simulink library "ammclib_bam_s32k11x"  (Simulink 9.0)
settings: Solver=ode45  StartTime=0.0  StopTime=10.0  RelTol=1e-3
undefined symbols (not defined in the file): f16A1, f16A2, f16B0, f16B1, f16B2, f16C1, f16CC1, f16CC1sc, f16CC1sc_D, f16CC1sc_Q, f16CC1scD, f16CC1scQ, f16CC2, f16CC2sc, f16CC2sc_D, f16CC2sc_Q, f16CC2scD, f16CC2scQ, f16DerivGain, f16EGain, f16FiltCoef, f16HystOff, f16HystOn, f16IGain, f16IntegGain, f16IntegGainFW, f16IntegGainQ, f16Kd, f16Kq, f16Limit, f16LowerLim, f16LowerLimit_D, f16LowerLimit_Q, f16ModIndex, f16OutValOff, f16OutValOn, f16PropGain, f16PropGainFW, f16PropGainQ, f16RampDown, f16RampUp, f16UGain, f16UpperLim, f16UpperLimit, f16UpperLimit_D, f16UpperLimit_Q, f16WIGain, f32A1, f32A2, f32B0, f32B1, f32B2, f32C1, f32CC1, f32CC1sc, f32CC1sc_D, f32CC1sc_Q, f32CC1scD, f32CC1scQ, f32CC2 ... (+71)
(part 5 of 7)

== system ammclib_bam_s32k11x/GFLIB/bam_f32/GFLIB_ControllerPIDpAW_F32 ==
  note: ---------------------------------------------------------------------------------------------------------------------------------------------------------------------------------------------------
  f32InErr : Inport
  f32UpperLimit : Inport  Port=2
  f32LowerLimit : Inport  Port=3
  Delay : Delay  DelayLength=1  InitialCondition=0
  Delay1 : Delay  DelayLength=1  InitialCondition=0
  Delay2 : Delay  DelayLength=1  InitialCondition=0
  GFLIB_ControllerPIDpAW_SF : S-Function  FunctionName=GFLIB_ControllerPIDpAW_SF_F32  Parameters=f32PropGain,s16PropGainShift,f32IntegGain,s16IntegGainShift,f32DerivGain,s16DerivGainShift,f32FiltCoef  SFunctionDeploymentMode=off  EnableBusSupport=off
  copyright : Subsystem
      mask Display: text(10,90,'FILE:');text(10,75,'DESRIPTION:');text(10,60,'COPYRIGHT:');text(10,45,'VERSION:');text(10,30,'DATE:')
  copyright2 : Subsystem
      mask Display: text(10,90,'GFLIB_ControllerPIDpAW_BAM_F32.mdl');text(10,75,'Parallel form of a standard PID controller with implemented anti-windup.');text(10,60,'NXP');text(10,45,'0.1');text(10,30,'21-Nov-2018');
  logo : Subsystem
      mask Display: image(imread('logo.jpg'))
  f32Out : Outport
  u16LimitFlag : Outport  Port=2
  wires:
  f32InErr/1 -> GFLIB_ControllerPIDpAW_SF/1
  f32UpperLimit/1 -> GFLIB_ControllerPIDpAW_SF/2
  f32LowerLimit/1 -> GFLIB_ControllerPIDpAW_SF/3
  Delay2/1 -> GFLIB_ControllerPIDpAW_SF/4
  Delay1/1 -> GFLIB_ControllerPIDpAW_SF/5
  Delay/1 -> GFLIB_ControllerPIDpAW_SF/6
  GFLIB_ControllerPIDpAW_SF/1 -> f32Out/1
  GFLIB_ControllerPIDpAW_SF/2 -> u16LimitFlag/1
  GFLIB_ControllerPIDpAW_SF/3 -> Delay2/1
  GFLIB_ControllerPIDpAW_SF/4 -> Delay1/1
  GFLIB_ControllerPIDpAW_SF/5 -> Delay/1

== system ammclib_bam_s32k11x/GFLIB/bam_f32/GFLIB_ControllerPIpAW_F32 ==
  note: ---------------------------------------------------------------------------------------------------------------------------------------------------------------------------------------------------
  f32InErr : Inport
  f32UpperLimit : Inport  Port=2
  f32LowerLimit : Inport  Port=3
  GFLIB_ControllerPIpAW_SF : S-Function  FunctionName=GFLIB_ControllerPIpAW_SF_F32  Parameters=f32PropGain,s16PropGainShift,f32IntegGain,s16IntegGainShift  SFunctionDeploymentMode=off  EnableBusSupport=off
  Unit_Delay_f32InK_1 : Delay  DelayLength=1  InitialCondition=0
  Unit_Delay_f32IntegPartK_1 : Delay  DelayLength=1  InitialCondition=0
  copyright : Subsystem
      mask Display: text(10,90,'FILE:');text(10,75,'DESRIPTION:');text(10,60,'COPYRIGHT:');text(10,45,'VERSION:');text(10,30,'DATE:')
  copyright2 : Subsystem
      mask Display: text(10,90,'GFLIB_ControllerPIpAW_BAM_F32.mdl');text(10,75,'Parallel form of a standard PI controller with implemented anti-windup.');text(10,60,'NXP');text(10,45,'0.1');text(10,30,'12-Jun-2015');
  logo : Subsystem
      mask Display: image(imread('logo.jpg'))
  f32Out : Outport
  u16LimitFlag : Outport  Port=2
  wires:
  GFLIB_ControllerPIpAW_SF/2 -> u16LimitFlag/1
  GFLIB_ControllerPIpAW_SF/1 -> f32Out/1
  f32LowerLimit/1 -> GFLIB_ControllerPIpAW_SF/3
  f32UpperLimit/1 -> GFLIB_ControllerPIpAW_SF/2
  f32InErr/1 -> GFLIB_ControllerPIpAW_SF/1
  Unit_Delay_f32IntegPartK_1/1 -> GFLIB_ControllerPIpAW_SF/5
  Unit_Delay_f32InK_1/1 -> GFLIB_ControllerPIpAW_SF/4
  GFLIB_ControllerPIpAW_SF/4 -> Unit_Delay_f32IntegPartK_1/1
  GFLIB_ControllerPIpAW_SF/3 -> Unit_Delay_f32InK_1/1

== system ammclib_bam_s32k11x/GFLIB/bam_f32/GFLIB_ControllerPIp_F32 ==
  note: ---------------------------------------------------------------------------------------------------------------------------------------------------------------------------------------------------
  f32InErr : Inport
  GFLIB_ControllerPIp_SF : S-Function  FunctionName=GFLIB_ControllerPIp_SF_F32  Parameters=f32PropGain,s16PropGainShift,f32IntegGain,s16IntegGainShift  SFunctionDeploymentMode=off  EnableBusSupport=off
  Unit_Delay_f32InIntegPartK_1 : UnitDelay  SampleTime=-1
  Unit_Delay_f32InK_1 : UnitDelay  SampleTime=-1
  copyright : Subsystem
      mask Display:
      | text(10,90,'FILE:');text(10,75,'DESRIPTION:')
      | text(10,60,'COPYRIGHT:')
      | text(10,45,'VERSION:')
      | text(10,30,'DATE:')
  copyright2 : Subsystem
      mask Display:
      | text(10,90,'GFLIB_ControllerPIp_BAM_F32.mdl');text(10,75,'Parallel form of a standard PI controller without implemented anti-windup.');text(10,60,'NXP')
      | text(10,45,'0.1');text(10,30,'20-Jan-2012');
  logo : Subsystem
      mask Display: image(imread('logo.jpg'))
  f32Out : Outport
  wires:
  GFLIB_ControllerPIp_SF/1 -> f32Out/1
  f32InErr/1 -> GFLIB_ControllerPIp_SF/1
  GFLIB_ControllerPIp_SF/3 -> Unit_Delay_f32InIntegPartK_1/1
  Unit_Delay_f32InIntegPartK_1/1 -> GFLIB_ControllerPIp_SF/3
  Unit_Delay_f32InK_1/1 -> GFLIB_ControllerPIp_SF/2
  GFLIB_ControllerPIp_SF/2 -> Unit_Delay_f32InK_1/1

== system ammclib_bam_s32k11x/GFLIB/bam_f32/GFLIB_ControllerPIrAW_F32 ==
  note: ---------------------------------------------------------------------------------------------------------------------------------------------------------------------------------------------------
  f32InErr : Inport
  f32UpperLimit : Inport  Port=2
  f32LowerLimit : Inport  Port=3
  GFLIB_ControllerPIrAW_SF : S-Function  FunctionName=GFLIB_ControllerPIrAW_SF_F32  Parameters=f32CC1,f32CC2,u16NShift  SFunctionDeploymentMode=off  EnableBusSupport=off
  Unit_Delay_f32Acc : Delay  DelayLength=1  InitialCondition=0
  Unit_Delay_f32InErrK1 : Delay  DelayLength=1  InitialCondition=0
  copyright : Subsystem
      mask Display: text(10,90,'FILE:');text(10,75,'DESRIPTION:');text(10,60,'COPYRIGHT:');text(10,45,'VERSION:');text(10,30,'DATE:')
  copyright2 : Subsystem
      mask Display: text(10,90,'GFLIB_ControllerPIrAW_BAM_F32.mdl');text(10,75,'Recurrent form of a standard PI controller with implemented anti-windup functionality.');text(10,60,'NXP');text(10,45,'0.1');text(10,30,'12-Jun-2015');
  logo : Subsystem
      mask Display: image(imread('logo.jpg'))
  f32Out : Outport
  wires:
  GFLIB_ControllerPIrAW_SF/1 -> f32Out/1
  f32LowerLimit/1 -> GFLIB_ControllerPIrAW_SF/3
  f32UpperLimit/1 -> GFLIB_ControllerPIrAW_SF/2
  f32InErr/1 -> GFLIB_ControllerPIrAW_SF/1
  GFLIB_ControllerPIrAW_SF/3 -> Unit_Delay_f32InErrK1/1
  GFLIB_ControllerPIrAW_SF/2 -> Unit_Delay_f32Acc/1
  Unit_Delay_f32InErrK1/1 -> GFLIB_ControllerPIrAW_SF/5
  Unit_Delay_f32Acc/1 -> GFLIB_ControllerPIrAW_SF/4

== system ammclib_bam_s32k11x/GFLIB/bam_f32/GFLIB_ControllerPIr_F32 ==
  note: ---------------------------------------------------------------------------------------------------------------------------------------------------------------------------------------------------
  f32InErr : Inport
  GFLIB_ControllerPIr_SF : S-Function  FunctionName=GFLIB_ControllerPIr_SF_F32  Parameters=f32CC1,f32CC2,u16NShift  SFunctionDeploymentMode=off  EnableBusSupport=off
  Unit_Delay_f32AccIn : UnitDelay  SampleTime=-1
  Unit_Delay_f32InErrK_1 : UnitDelay  SampleTime=-1
  copyright : Subsystem
      mask Display:
      | text(10,90,'FILE:');text(10,75,'DESRIPTION:')
      | text(10,60,'COPYRIGHT:')
      | text(10,45,'VERSION:')
      | text(10,30,'DATE:')
  copyright2 : Subsystem
      mask Display:
      | text(10,90,'GFLIB_ControllerPIr_BAM_F32.mdl');text(10,75,'Recurrent form of a standard PI controller without implemented anti-windup.');text(10,60,'NXP')
      | text(10,45,'0.1');text(10,30,'20-Jan-2012');
  logo : Subsystem
      mask Display: image(imread('logo.jpg'))
  f32Out : Outport
  wires:
  GFLIB_ControllerPIr_SF/1 -> f32Out/1
  f32InErr/1 -> GFLIB_ControllerPIr_SF/1
  Unit_Delay_f32InErrK_1/1 -> GFLIB_ControllerPIr_SF/3
  Unit_Delay_f32AccIn/1 -> GFLIB_ControllerPIr_SF/2
  GFLIB_ControllerPIr_SF/3 -> Unit_Delay_f32InErrK_1/1
  GFLIB_ControllerPIr_SF/2 -> Unit_Delay_f32AccIn/1

== system ammclib_bam_s32k11x/GFLIB/bam_f32/GFLIB_Cos_F32 ==
  note: ---------------------------------------------------------------------------------------------------------------------------------------------------------------------------------------------------
  f32In : Inport
  GFLIB_Cos_SF : S-Function  FunctionName=GFLIB_Cos_SF_F32  SFunctionDeploymentMode=off  EnableBusSupport=off
  copyright : Subsystem
      mask Display: text(10,90,'FILE:');text(10,75,'DESRIPTION:')text(10,60,'COPYRIGHT:')text(10,45,'VERSION:')text(10,30,'DATE:')
  copyright2 : Subsystem
      mask Display: text(10,90,'GFLIB_Cos_BAM_F32.mdl');text(10,75,'Cosine transformation');text(10,60,'NXP')text(10,45,'0.1');text(10,30,'13-Sep-2011');
  logo : Subsystem
      mask Display: image(imread('logo.jpg'))
  f32Out : Outport
  wires:
  GFLIB_Cos_SF/1 -> f32Out/1
  f32In/1 -> GFLIB_Cos_SF/1

== system ammclib_bam_s32k11x/GFLIB/bam_f32/GFLIB_Hyst_F32 ==
  note: ---------------------------------------------------------------------------------------------------------------------------------------------------------------------------------------------------
  f32In : Inport
  GFLIB_Hyst_SF_F32 : S-Function  FunctionName=GFLIB_Hyst_SF_F32  Parameters=f32HystOn,f32HystOff,f32OutValOn,f32OutValOff  SFunctionDeploymentMode=off  EnableBusSupport=off
  Unit_Delay_f32InState : UnitDelay  SampleTime=-1
  copyright : Subsystem
      mask Display:
      | text(10,90,'FILE:');text(10,75,'DESRIPTION:')
      | text(10,60,'COPYRIGHT:')
      | text(10,45,'VERSION:')
      | text(10,30,'DATE:')
  copyright2 : Subsystem
      mask Display:
      | text(10,90,'GFLIB_Hyst_BAM_F32.mdl');text(10,75,'Hysteresis function.');text(10,60,'NXP')
      | text(10,45,'0.1');text(10,30,'09-Apr-2014');
  logo : Subsystem
      mask Display: image(imread('logo.jpg'))
  f32Out : Outport
  wires:
  GFLIB_Hyst_SF_F32/1 -> f32Out/1
  f32In/1 -> GFLIB_Hyst_SF_F32/1
  Unit_Delay_f32InState/1 -> GFLIB_Hyst_SF_F32/2
  GFLIB_Hyst_SF_F32/2 -> Unit_Delay_f32InState/1

== system ammclib_bam_s32k11x/GFLIB/bam_f32/GFLIB_IntegratorTR_F32 ==
  note: ---------------------------------------------------------------------------------------------------------------------------------------------------------------------------------------------------
  f32In : Inport
  GFLIB_IntegratorTR_SF : S-Function  FunctionName=GFLIB_IntegratorTR_SF_F32  Parameters=f32C1,u16NShift  SFunctionDeploymentMode=off  EnableBusSupport=off
  Unit_Delay_f32InAcc : UnitDelay  SampleTime=-1
  Unit_Delay_f32InK_1 : UnitDelay  SampleTime=-1
  copyright : Subsystem
      mask Display:
      | text(10,90,'FILE:');text(10,75,'DESRIPTION:')
      | text(10,60,'COPYRIGHT:')
      | text(10,45,'VERSION:')
      | text(10,30,'DATE:')
  copyright2 : Subsystem
      mask Display:
      | text(10,90,'GFLIB_IntegratorTR_BAM_F32.mdl');text(10,75,'Discrete integrator transformed from linear model using Billinear (trapezoidal) transformation.');text(10,60,'NXP')
      | text(10,45,'0.1');text(10,30,'16-Jan-2012');
  logo : Subsystem
      mask Display: image(imread('logo.jpg'))
  f32Out : Outport
  wires:
  GFLIB_IntegratorTR_SF/1 -> f32Out/1
  f32In/1 -> GFLIB_IntegratorTR_SF/1
  GFLIB_IntegratorTR_SF/3 -> Unit_Delay_f32InK_1/1
  Unit_Delay_f32InK_1/1 -> GFLIB_IntegratorTR_SF/3
  Unit_Delay_f32InAcc/1 -> GFLIB_IntegratorTR_SF/2
  GFLIB_IntegratorTR_SF/2 -> Unit_Delay_f32InAcc/1

== system ammclib_bam_s32k11x/GFLIB/bam_f32/GFLIB_Limit_F32 ==
  note: ---------------------------------------------------------------------------------------------------------------------------------------------------------------------------------------------------
  f32In : Inport
  GFLIB_Limit_SF_F32 : S-Function  FunctionName=GFLIB_Limit_SF_F32  Parameters=f32UpperLimit,f32LowerLim  SFunctionDeploymentMode=off  EnableBusSupport=off
  copyright : Subsystem
      mask Display:
      | text(10,90,'FILE:');text(10,75,'DESRIPTION:')
      | text(10,60,'COPYRIGHT:')
      | text(10,45,'VERSION:')
      | text(10,30,'DATE:')
      | text(10,15,'AUTHOR:')
  copyright2 : Subsystem
      mask Display:
      | text(10,90,'GFLIB_Limit_BAM_F32.mdl');text(10,75,'Limit function');text(10,60,'NXP')
      | text(10,45,'0.1');text(10,30,'03-Jul-2011');text(10,15,'');
  logo : Subsystem
      mask Display: image(imread('logo.jpg'))
  f32Out : Outport
  wires:
  GFLIB_Limit_SF_F32/1 -> f32Out/1
  f32In/1 -> GFLIB_Limit_SF_F32/1

== system ammclib_bam_s32k11x/GFLIB/bam_f32/GFLIB_LowerLimit_F32 ==
  note: ---------------------------------------------------------------------------------------------------------------------------------------------------------------------------------------------------
  f32In : Inport
  GFLIB_LowerLimit_SF_F32 : S-Function  FunctionName=GFLIB_LowerLimit_SF_F32  Parameters=f32LowerLim  SFunctionDeploymentMode=off  EnableBusSupport=off
  copyright : Subsystem
      mask Display:
      | text(10,90,'FILE:');text(10,75,'DESRIPTION:')
      | text(10,60,'COPYRIGHT:')
      | text(10,45,'VERSION:')
      | text(10,30,'DATE:')
  copyright2 : Subsystem
      mask Display:
      | text(10,90,'GFLIB_LowerLimit_BAM_F32.mdl');text(10,75,'Lower limit function.');text(10,60,'Freescale')
      | text(10,45,'0.1');text(10,30,'13-Sep-2011');
  logo : Subsystem
      mask Display: image(imread('logo.jpg'))
  f32Out : Outport
  wires:
  GFLIB_LowerLimit_SF_F32/1 -> f32Out/1
  f32In/1 -> GFLIB_LowerLimit_SF_F32/1

== system ammclib_bam_s32k11x/GFLIB/bam_f32/GFLIB_Lut1D_F32 ==
  note: ---------------------------------------------------------------------------------------------------------------------------------------------------------------------------------------------------
  f32In : Inport
  GFLIB_Lut1D_SF : S-Function  FunctionName=GFLIB_Lut1D_SF_F32  Parameters=u32ShamOffset,pf32Table,s32MidIdx  SFunctionDeploymentMode=off  EnableBusSupport=off
  copyright : Subsystem
      mask Display:
      | text(10,90,'FILE:');text(10,75,'DESRIPTION:')
      | text(10,60,'COPYRIGHT:')
      | text(10,45,'VERSION:')
      | text(10,30,'DATE:')
  copyright2 : Subsystem
      mask Display:
      | text(10,90,'GFLIB_Lut1D_BAM_F32.mdl');text(10,75,'One dimensional Look-up table function');text(10,60,'Freescale')
      | text(10,45,'0.1');text(10,30,'17-Jun-2013');
  logo : Subsystem
      mask Display: image(imread('logo.jpg'))
  f32Out : Outport
  wires:
  f32In/1 -> GFLIB_Lut1D_SF/1
  GFLIB_Lut1D_SF/1 -> f32Out/1

== system ammclib_bam_s32k11x/GFLIB/bam_f32/GFLIB_Lut2D_F32 ==
  note: ---------------------------------------------------------------------------------------------------------------------------------------------------------------------------------------------------
  f32In1 : Inport
  f32In2 : Inport  Port=2
  GFLIB_Lut2D_SF : S-Function  FunctionName=GFLIB_Lut2D_SF_F32  Parameters=u32ShamOffset1,u32ShamOffset2,pf32Table,s32MidIdx  SFunctionDeploymentMode=off  EnableBusSupport=off
  copyright : Subsystem
      mask Display:
      | text(10,90,'FILE:');text(10,75,'DESRIPTION:')
      | text(10,60,'COPYRIGHT:')
      | text(10,45,'VERSION:')
      | text(10,30,'DATE:')
  copyright2 : Subsystem
      mask Display:
      | text(10,90,'GFLIB_Lut2D_BAM_F32.mdl');text(10,75,'Two dimensional Look-up table function');text(10,60,'NXP')
      | text(10,45,'0.1');text(10,30,'17-Jun-2013');
  logo : Subsystem
      mask Display: image(imread('logo.jpg'))
  f32Out : Outport
  wires:
  GFLIB_Lut2D_SF/1 -> f32Out/1
  f32In2/1 -> GFLIB_Lut2D_SF/2
  f32In1/1 -> GFLIB_Lut2D_SF/1

== system ammclib_bam_s32k11x/GFLIB/bam_f32/GFLIB_Ramp_F32 ==
  note: ---------------------------------------------------------------------------------------------------------------------------------------------------------------------------------------------------
  f32In : Inport
  GFLIB_Ramp_SF_F32 : S-Function  FunctionName=GFLIB_Ramp_SF_F32  Parameters=f32RampUp,f32RampDown  SFunctionDeploymentMode=off  EnableBusSupport=off
  Unit_Delay_f32InState : UnitDelay  SampleTime=-1
  copyright : Subsystem
      mask Display:
      | text(10,90,'FILE:');text(10,75,'DESRIPTION:')
      | text(10,60,'COPYRIGHT:')
      | text(10,45,'VERSION:')
      | text(10,30,'DATE:')
      | text(10,15,'AUTHOR:')
  copyright2 : Subsystem
      mask Display:
      | text(10,90,'GFLIB_Ramp_BAM_F32.mdl');text(10,75,'Rate of change limiter - Ramp function.');text(10,60,'NXP')
      | text(10,45,'0.1');text(10,30,'08-Apr-2014');text(10,15,'');
  logo : Subsystem
      mask Display: image(imread('logo.jpg'))
  f32Out : Outport
  wires:
  GFLIB_Ramp_SF_F32/1 -> f32Out/1
  f32In/1 -> GFLIB_Ramp_SF_F32/1
  Unit_Delay_f32InState/1 -> GFLIB_Ramp_SF_F32/2
  GFLIB_Ramp_SF_F32/2 -> Unit_Delay_f32InState/1

== system ammclib_bam_s32k11x/GFLIB/bam_f32/GFLIB_Sign_F32 ==
  note: ---------------------------------------------------------------------------------------------------------------------------------------------------------------------------------------------------
  f32In : Inport
  GFLIB_Sign_SF_F32 : S-Function  FunctionName=GFLIB_Sign_SF_F32  SFunctionDeploymentMode=off  EnableBusSupport=off
  copyright : Subsystem
      mask Display:
      | text(10,90,'FILE:');text(10,75,'DESRIPTION:')
      | text(10,60,'COPYRIGHT:')
      | text(10,45,'VERSION:')
      | text(10,30,'DATE:')
  copyright2 : Subsystem
      mask Display:
      | text(10,90,'GFLIB_Sign_BAM_F32.mdl');text(10,75,'Sign function.');text(10,60,'NXP')
      | text(10,45,'0.1');text(10,30,'26-Aug-2011');
  logo : Subsystem
      mask Display: image(imread('logo.jpg'))
  f32Out : Outport
  wires:
  GFLIB_Sign_SF_F32/1 -> f32Out/1
  f32In/1 -> GFLIB_Sign_SF_F32/1

== system ammclib_bam_s32k11x/GFLIB/bam_f32/GFLIB_SinCos_F32 ==
  note: ---------------------------------------------------------------------------------------------------------------------------------------------------------------------------------------------------
  f32In : Inport
  GFLIB_SinCos_SF : S-Function  FunctionName=GFLIB_SinCos_SF_F32  SFunctionDeploymentMode=off  EnableBusSupport=off
  copyright : Subsystem
      mask Display: text(10,90,'FILE:');text(10,75,'DESRIPTION:');text(10,60,'COPYRIGHT:');text(10,45,'VERSION:');text(10,30,'DATE:')
  copyright2 : Subsystem
      mask Display: text(10,90,'GFLIB_SinCos_BAM_F32.mdl');text(10,75,'Sine and Cosine transformation');text(10,60,'Freescale');text(10,45,'0.1');text(10,30,'27-Sep-2015');
  logo : Subsystem
      mask Display: image(imread('logo.jpg'))
  f32SinOut : Outport
  f32CosOut : Outport  Port=2
  wires:
  GFLIB_SinCos_SF/2 -> f32CosOut/1
  GFLIB_SinCos_SF/1 -> f32SinOut/1
  f32In/1 -> GFLIB_SinCos_SF/1

== system ammclib_bam_s32k11x/GFLIB/bam_f32/GFLIB_Sin_F32 ==
  note: ---------------------------------------------------------------------------------------------------------------------------------------------------------------------------------------------------
  f32In : Inport
  GFLIB_Sin_SF : S-Function  FunctionName=GFLIB_Sin_SF_F32  SFunctionDeploymentMode=off  EnableBusSupport=off
  copyright : Subsystem
      mask Display:
      | text(10,90,'FILE:');text(10,75,'DESRIPTION:')
      | text(10,60,'COPYRIGHT:')
      | text(10,45,'VERSION:')
      | text(10,30,'DATE:')
  copyright2 : Subsystem
      mask Display:
      | text(10,90,'GFLIB_Sin_BAM_F32.mdl');text(10,75,'Sine transformation');text(10,60,'NXP')
      | text(10,45,'0.1');text(10,30,'13-Sep-2011');
  logo : Subsystem
      mask Display: image(imread('logo.jpg'))
  f32Out : Outport
  wires:
  GFLIB_Sin_SF/1 -> f32Out/1
  f32In/1 -> GFLIB_Sin_SF/1

== system ammclib_bam_s32k11x/GFLIB/bam_f32/GFLIB_Sqrt_F32 ==
  note: ---------------------------------------------------------------------------------------------------------------------------------------------------------------------------------------------------
  f32In : Inport
  GFLIB_Sqrt_SF_F32 : S-Function  FunctionName=GFLIB_Sqrt_SF_F32  SFunctionDeploymentMode=off  EnableBusSupport=off
  copyright : Subsystem
      mask Display:
      | text(10,90,'FILE:');text(10,75,'DESRIPTION:')
      | text(10,60,'COPYRIGHT:')
      | text(10,45,'VERSION:')
      | text(10,30,'DATE:')
  copyright2 : Subsystem
      mask Display:
      | text(10,90,'GFLIB_Sqrt_BAM_F32.mdl');text(10,75,'Square root approximation.');text(10,60,'Freescale')
      | text(10,45,'0.1');text(10,30,'12-Sep-2011');
  logo : Subsystem
      mask Display: image(imread('logo.jpg'))
  f32Out : Outport
  wires:
  GFLIB_Sqrt_SF_F32/1 -> f32Out/1
  f32In/1 -> GFLIB_Sqrt_SF_F32/1

== system ammclib_bam_s32k11x/GFLIB/bam_f32/GFLIB_Tan_F32 ==
  note: ---------------------------------------------------------------------------------------------------------------------------------------------------------------------------------------------------
  f32In : Inport
  GFLIB_Tan_SF : S-Function  FunctionName=GFLIB_Tan_SF_F32  SFunctionDeploymentMode=off  EnableBusSupport=off
  copyright : Subsystem
      mask Display: text(10,90,'FILE:');text(10,75,'DESRIPTION:')text(10,60,'COPYRIGHT:')text(10,45,'VERSION:')text(10,30,'DATE:')
  copyright2 : Subsystem
      mask Display: text(10,90,'GFLIB_Tan_BAM_F32.mdl');text(10,75,'Tangent transformation');text(10,60,'NXP')text(10,45,'0.1');text(10,30,'13-Sep-2011');
  logo : Subsystem
      mask Display: image(imread('logo.jpg'))
  f32Out : Outport
  wires:
  GFLIB_Tan_SF/1 -> f32Out/1
  f32In/1 -> GFLIB_Tan_SF/1

== system ammclib_bam_s32k11x/GFLIB/bam_f32/GFLIB_UpperLimit_F32 ==
  note: ---------------------------------------------------------------------------------------------------------------------------------------------------------------------------------------------------
  f32In : Inport
  GFLIB_UpperLimit_SF_F32 : S-Function  FunctionName=GFLIB_UpperLimit_SF_F32  Parameters=f32UpperLim  SFunctionDeploymentMode=off  EnableBusSupport=off
  copyright : Subsystem
      mask Display:
      | text(10,90,'FILE:');text(10,75,'DESRIPTION:')
      | text(10,60,'COPYRIGHT:')
      | text(10,45,'VERSION:')
      | text(10,30,'DATE:')
  copyright2 : Subsystem
      mask Display:
      | text(10,90,'GFLIB_UpperLimit_BAM_F32.mdl');text(10,75,'Upper limit function.');text(10,60,'Freescale')
      | text(10,45,'0.1');text(10,30,'13-Sep-2011');
  logo : Subsystem
      mask Display: image(imread('logo.jpg'))
  f32Out : Outport
  wires:
  GFLIB_UpperLimit_SF_F32/1 -> f32Out/1
  f32In/1 -> GFLIB_UpperLimit_SF_F32/1

== system ammclib_bam_s32k11x/GFLIB/bam_f32/GFLIB_VMin_F32 ==
  note: ---------------------------------------------------------------------------------------------------------------------------------------------------------------------------------------------------
  InputVector : Inport
  GFLIB_VMin_SF : S-Function  FunctionName=GFLIB_VMin_SF_F32  Parameters=N  SFunctionDeploymentMode=off  EnableBusSupport=off
  Gain : Gain  Gain=[eye(N) zeros(N,256-N)]'  Multiplication=Matrix(K*u)  OutDataTypeStr=int32
  copyright : Subsystem
      mask Display: text(10,90,'FILE:');text(10,75,'DESRIPTION:');text(10,60,'COPYRIGHT:');text(10,45,'VERSION:');text(10,30,'DATE:')
  copyright2 : Subsystem
      mask Display: text(10,90,'GFLIB_VMin_BAM_F32.mdl');text(10,75,'Vector minimum');text(10,60,'NXP');text(10,45,'1.0');text(10,30,'18-Jan-2018');
  logo : Subsystem
      mask Display: image(imread('logo.jpg'))
  IndexOfMinimum : Outport
  wires:
  InputVector/1 -> Gain/1
  Gain/1 -> GFLIB_VMin_SF/1
  GFLIB_VMin_SF/1 -> IndexOfMinimum/1

== system ammclib_bam_s32k11x/GFLIB/bam_f32/GFLIB_VectorLimit_F32 ==
  note: ---------------------------------------------------------------------------------------------------------------------------------------------------------------------------------------------------
  f32InVec1 : Inport
  f32InVec2 : Inport  Port=2
  GFLIB_VectorLimit_SF_F32 : S-Function  FunctionName=GFLIB_VectorLimit_SF_F32  Parameters=f32Limit  SFunctionDeploymentMode=off  EnableBusSupport=off
  copyright : Subsystem
      mask Display:
      | text(10,90,'FILE:');text(10,75,'DESRIPTION:')
      | text(10,60,'COPYRIGHT:')
      | text(10,45,'VERSION:')
      | text(10,30,'DATE:')
      | text(10,15,'AUTHOR:')
  copyright2 : Subsystem
      mask Display:
      | text(10,90,'GFLIB_VectorLimit_BAM_F32.mdl');text(10,75,'Vector limit function');text(10,60,'Freescale')
      | text(10,45,'0.1');text(10,30,'15-Sep-2011');text(10,15,'');
  logo : Subsystem
      mask Display: image(imread('logo.jpg'))
  f32OutVec1 : Outport
  f32OutVec2 : Outport  Port=2
  bFlag : Outport  Port=3
  wires:
  GFLIB_VectorLimit_SF_F32/3 -> bFlag/1
  GFLIB_VectorLimit_SF_F32/2 -> f32OutVec2/1
  f32InVec2/1 -> GFLIB_VectorLimit_SF_F32/2
  GFLIB_VectorLimit_SF_F32/1 -> f32OutVec1/1
  f32InVec1/1 -> GFLIB_VectorLimit_SF_F32/1

== system ammclib_bam_s32k11x/GMCLIB/bam_f16/GMCLIB_ClarkInv_F16 ==
  note: ---------------------------------------------------------------------------------------------------------------------------------------------------------------------------------------------------
  f16Alpha : Inport
  f16Beta : Inport  Port=2
  GMCLIB_ClarkInv_SF_F16 : S-Function  FunctionName=GMCLIB_ClarkInv_SF_F16  SFunctionDeploymentMode=off  EnableBusSupport=off
  copyright : Subsystem
      mask Display:
      | text(10,90,'FILE:');text(10,75,'DESRIPTION:')
      | text(10,60,'COPYRIGHT:')
      | text(10,45,'VERSION:')
      | text(10,30,'DATE:')
  copyright2 : Subsystem
      mask Display:
      | text(10,90,'GMCLIB_ClarkInv_BAM_F16.mdl');text(10,75,'Inverse Clarke transformation');text(10,60,'NXP')
      | text(10,45,'0.1');text(10,30,'30-Aug-2011');
  logo : Subsystem
      mask Display: image(imread('logo.jpg'))
  f16A : Outport
  f16B : Outport  Port=2
  f16C : Outport  Port=3
  wires:
  GMCLIB_ClarkInv_SF_F16/3 -> f16C/1
  GMCLIB_ClarkInv_SF_F16/2 -> f16B/1
  GMCLIB_ClarkInv_SF_F16/1 -> f16A/1
  f16Beta/1 -> GMCLIB_ClarkInv_SF_F16/2
  f16Alpha/1 -> GMCLIB_ClarkInv_SF_F16/1

== system ammclib_bam_s32k11x/GMCLIB/bam_f16/GMCLIB_Clark_F16 ==
  note: ---------------------------------------------------------------------------------------------------------------------------------------------------------------------------------------------------
  f16A : Inport
  f16B : Inport  Port=2
  f16C : Inport  Port=3
  GMCLIB_Clark_SF_F16 : S-Function  FunctionName=GMCLIB_Clark_SF_F16  SFunctionDeploymentMode=off  EnableBusSupport=off
  copyright : Subsystem
      mask Display:
      | text(10,90,'FILE:');text(10,75,'DESRIPTION:')
      | text(10,60,'COPYRIGHT:')
      | text(10,45,'VERSION:')
      | text(10,30,'DATE:')
  copyright2 : Subsystem
      mask Display:
      | text(10,90,'GMCLIB_Clark_BAM_F16.mdl');text(10,75,'Clarke transformation.');text(10,60,'NXP')
      | text(10,45,'0.1');text(10,30,'29-Aug-2011');
  logo : Subsystem
      mask Display: image(imread('logo.jpg'))
  f16Alpha : Outport
  f16Beta : Outport  Port=2
  wires:
  GMCLIB_Clark_SF_F16/2 -> f16Beta/1
  GMCLIB_Clark_SF_F16/1 -> f16Alpha/1
  f16C/1 -> GMCLIB_Clark_SF_F16/3
  f16B/1 -> GMCLIB_Clark_SF_F16/2
  f16A/1 -> GMCLIB_Clark_SF_F16/1

== system ammclib_bam_s32k11x/GMCLIB/bam_f16/GMCLIB_DecouplingPMSM_F16 ==
  note: ---------------------------------------------------------------------------------------------------------------------------------------------------------------------------------------------------
  f16Ud : Inport
  f16Uq : Inport  Port=2
  f16Id : Inport  Port=3
  f16Iq : Inport  Port=4
  f16AngVel : Inport  Port=5
  GMCLIB_DecouplingPMSM_SF_F16 : S-Function  FunctionName=GMCLIB_DecouplingPMSM_SF_F16  Parameters=f16Kd,s16KdShift,f16Kq,s16KqShift  SFunctionDeploymentMode=off  EnableBusSupport=off
  copyright : Subsystem
      mask Display:
      | text(10,90,'FILE:');text(10,75,'DESRIPTION:')
      | text(10,60,'COPYRIGHT:')
      | text(10,45,'VERSION:')
      | text(10,30,'DATE:')
  copyright2 : Subsystem
      mask Display:
      | text(10,90,'GMCLIB_DecouplingPMSM_BAM_F16.mdl');text(10,75,'Decoupling of d and q axis of PMSM model.');text(10,60,'NXP')
      | text(10,45,'0.1');text(10,30,'14-Sep-2011');
  logo : Subsystem
      mask Display: image(imread('logo.jpg'))
  f16UdDec : Outport
  f16UqDec : Outport  Port=2
  wires:
  GMCLIB_DecouplingPMSM_SF_F16/2 -> f16UqDec/1
  GMCLIB_DecouplingPMSM_SF_F16/1 -> f16UdDec/1
  f16AngVel/1 -> GMCLIB_DecouplingPMSM_SF_F16/5
  f16Iq/1 -> GMCLIB_DecouplingPMSM_SF_F16/4
  f16Id/1 -> GMCLIB_DecouplingPMSM_SF_F16/3
  f16Uq/1 -> GMCLIB_DecouplingPMSM_SF_F16/2
  f16Ud/1 -> GMCLIB_DecouplingPMSM_SF_F16/1

== system ammclib_bam_s32k11x/GMCLIB/bam_f16/GMCLIB_ElimDcBusRip_F16 ==
  note: ---------------------------------------------------------------------------------------------------------------------------------------------------------------------------------------------------
  f16Alpha : Inport
  f16Beta : Inport  Port=2
  f16ArgDcBusMsr : Inport  Port=3
  GMCLIB_ElimDcBusRip_SF : S-Function  FunctionName=GMCLIB_ElimDcBusRip_SF_F16  Parameters=f16ModIndex  SFunctionDeploymentMode=off  EnableBusSupport=off
  copyright : Subsystem
      mask Display: text(10,90,'FILE:');text(10,75,'DESRIPTION:');text(10,60,'COPYRIGHT:');text(10,45,'VERSION:');text(10,30,'DATE:')
  copyright2 : Subsystem
      mask Display: text(10,90,'GMCLIB_ElimDcBusRip_BAM_F16.mdl');text(10,75,'DC Bus voltage ripple elimination function.');text(10,60,'NXP');text(10,45,'0.1');text(10,30,'12-Jun-2015');
  logo : Subsystem
      mask Display: image(imread('logo.jpg'))
  f16AlphaOut : Outport
  f16BetaOut : Outport  Port=2
  wires:
  GMCLIB_ElimDcBusRip_SF/2 -> f16BetaOut/1
  GMCLIB_ElimDcBusRip_SF/1 -> f16AlphaOut/1
  f16ArgDcBusMsr/1 -> GMCLIB_ElimDcBusRip_SF/3
  f16Beta/1 -> GMCLIB_ElimDcBusRip_SF/2
  f16Alpha/1 -> GMCLIB_ElimDcBusRip_SF/1

== system ammclib_bam_s32k11x/GMCLIB/bam_f16/GMCLIB_ParkInv_F16 ==
  note: ---------------------------------------------------------------------------------------------------------------------------------------------------------------------------------------------------
  f16D : Inport
  f16Q : Inport  Port=2
  f16Sin : Inport  Port=3
  f16Cos : Inport  Port=4
  GMCLIB_ParkInv_SF : S-Function  FunctionName=GMCLIB_ParkInv_SF_F16  SFunctionDeploymentMode=off  EnableBusSupport=off
  copyright : Subsystem
      mask Display:
      | text(10,90,'FILE:');text(10,75,'DESRIPTION:')
      | text(10,60,'COPYRIGHT:')
      | text(10,45,'VERSION:')
      | text(10,30,'DATE:')
  copyright2 : Subsystem
      mask Display:
      | text(10,90,'GMCLIB_ParkInv_BAM_F16.mdl');text(10,75,'Inverse Park transformation.');text(10,60,'Freescale')
      | text(10,45,'0.1');text(10,30,'19-Sep-2011');
  logo : Subsystem
      mask Display: image(imread('logo.jpg'))
  f16Alpha : Outport
  f16Beta : Outport  Port=2
  wires:
  GMCLIB_ParkInv_SF/2 -> f16Beta/1
  GMCLIB_ParkInv_SF/1 -> f16Alpha/1
  f16Cos/1 -> GMCLIB_ParkInv_SF/4
  f16Sin/1 -> GMCLIB_ParkInv_SF/3
  f16Q/1 -> GMCLIB_ParkInv_SF/2
  f16D/1 -> GMCLIB_ParkInv_SF/1

== system ammclib_bam_s32k11x/GMCLIB/bam_f16/GMCLIB_Park_F16 ==
  note: ---------------------------------------------------------------------------------------------------------------------------------------------------------------------------------------------------
  f16Alpha : Inport
  f16Beta : Inport  Port=2
  f16Sin : Inport  Port=3
  f16Cos : Inport  Port=4
  GMCLIB_Park_SF : S-Function  FunctionName=GMCLIB_Park_SF_F16  SFunctionDeploymentMode=off  EnableBusSupport=off
  copyright : Subsystem
      mask Display:
      | text(10,90,'FILE:');text(10,75,'DESRIPTION:')
      | text(10,60,'COPYRIGHT:')
      | text(10,45,'VERSION:')
      | text(10,30,'DATE:')
  copyright2 : Subsystem
      mask Display:
      | text(10,90,'GMCLIB_Park_BAM_F16.mdl');text(10,75,'Park transformation.');text(10,60,'NXP')
      | text(10,45,'0.1');text(10,30,'19-Sep-2011');
  logo : Subsystem
      mask Display: image(imread('logo.jpg'))
  f16D : Outport
  f16Q : Outport  Port=2
  wires:
  GMCLIB_Park_SF/2 -> f16Q/1
  GMCLIB_Park_SF/1 -> f16D/1
  f16Cos/1 -> GMCLIB_Park_SF/4
  f16Sin/1 -> GMCLIB_Park_SF/3
  f16Beta/1 -> GMCLIB_Park_SF/2
  f16Alpha/1 -> GMCLIB_Park_SF/1

== system ammclib_bam_s32k11x/GMCLIB/bam_f16/GMCLIB_PwmIct_F16 ==
  note: ---------------------------------------------------------------------------------------------------------------------------------------------------------------------------------------------------
  f16In1 : Inport
  f16In2 : Inport  Port=2
  GMCLIB_PwmIct_SF : S-Function  FunctionName=GMCLIB_PwmIct_SF_F16  SFunctionDeploymentMode=off  EnableBusSupport=off
  copyright : Subsystem
      mask Display: text(10,90,'FILE:');text(10,75,'DESRIPTION:');text(10,60,'COPYRIGHT:');text(10,45,'VERSION:');text(10,30,'DATE:')
  copyright2 : Subsystem
      mask Display: text(10,90,'GMCLIB_PwmIct_BAM_F16.mdl');text(10,75,'General Sinusoidal PWM.');text(10,60,'NXP');text(10,45,'1.0');text(10,30,'05-Apr-2019');
  logo : Subsystem
      mask Display: image(imread('logo.jpg'))
  f16Out1 : Outport
  f16Out2 : Outport  Port=2
  f16Out3 : Outport  Port=3
  u16Sector : Outport  Port=4
  wires:
  f16In1/1 -> GMCLIB_PwmIct_SF/1
  f16In2/1 -> GMCLIB_PwmIct_SF/2
  GMCLIB_PwmIct_SF/1 -> f16Out1/1
  GMCLIB_PwmIct_SF/2 -> f16Out2/1
  GMCLIB_PwmIct_SF/3 -> f16Out3/1
  GMCLIB_PwmIct_SF/4 -> u16Sector/1

== system ammclib_bam_s32k11x/GMCLIB/bam_f16/GMCLIB_SvmStd_F16 ==
  note: ---------------------------------------------------------------------------------------------------------------------------------------------------------------------------------------------------
  f16In1 : Inport
  f16In2 : Inport  Port=2
  GMCLIB_SvmStd_SF : S-Function  FunctionName=GMCLIB_SvmStd_SF_F16  SFunctionDeploymentMode=off  EnableBusSupport=off
  copyright : Subsystem
      mask Display:
      | text(10,90,'FILE:');text(10,75,'DESRIPTION:')
      | text(10,60,'COPYRIGHT:')
      | text(10,45,'VERSION:')
      | text(10,30,'DATE:')
  copyright2 : Subsystem
      mask Display:
      | text(10,90,'GMCLIB_SvmStd_BAM_F16.mdl');text(10,75,'Standard Space Vector Modulation.');text(10,60,'NXP')
      | text(10,45,'0.1');text(10,30,'26-Sep-2011');
  logo : Subsystem
      mask Display: image(imread('logo.jpg'))
  f16Out1 : Outport
  f16Out2 : Outport  Port=2
  f16Out3 : Outport  Port=3
  u16Sector : Outport  Port=4
  wires:
  GMCLIB_SvmStd_SF/4 -> u16Sector/1
  GMCLIB_SvmStd_SF/3 -> f16Out3/1
  GMCLIB_SvmStd_SF/2 -> f16Out2/1
  GMCLIB_SvmStd_SF/1 -> f16Out1/1
  f16In2/1 -> GMCLIB_SvmStd_SF/2
  f16In1/1 -> GMCLIB_SvmStd_SF/1

== system ammclib_bam_s32k11x/GMCLIB/bam_f16/GMCLIB_SvmU0n_F16 ==
  note: ---------------------------------------------------------------------------------------------------------------------------------------------------------------------------------------------------
  f16In1 : Inport
  f16In2 : Inport  Port=2
  GMCLIB_SvmU0n_SF : S-Function  FunctionName=GMCLIB_SvmU0n_SF_F16  SFunctionDeploymentMode=off  EnableBusSupport=off
  copyright : Subsystem
      mask Display: text(10,90,'FILE:');text(10,75,'DESRIPTION:');text(10,60,'COPYRIGHT:');text(10,45,'VERSION:');text(10,30,'DATE:')
  copyright2 : Subsystem
      mask Display: text(10,90,'GMCLIB_SvmU0n_BAM_F16.mdl');text(10,75,'Standard Space Vector Modulation.');text(10,60,'NXP');text(10,45,'0.1');text(10,30,'02-Apr-2019');
  logo : Subsystem
      mask Display: image(imread('logo.jpg'))
  f16Out1 : Outport
  f16Out2 : Outport  Port=2
  f16Out3 : Outport  Port=3
  u16Sector : Outport  Port=4
  wires:
  f16In1/1 -> GMCLIB_SvmU0n_SF/1
  f16In2/1 -> GMCLIB_SvmU0n_SF/2
  GMCLIB_SvmU0n_SF/1 -> f16Out1/1
  GMCLIB_SvmU0n_SF/2 -> f16Out2/1
  GMCLIB_SvmU0n_SF/3 -> f16Out3/1
  GMCLIB_SvmU0n_SF/4 -> u16Sector/1

== system ammclib_bam_s32k11x/GMCLIB/bam_f32/GMCLIB_ClarkInv_F32 ==
  note: ---------------------------------------------------------------------------------------------------------------------------------------------------------------------------------------------------
  f32Alpha : Inport
  f32Beta : Inport  Port=2
  GMCLIB_ClarkInv_SF_F32 : S-Function  FunctionName=GMCLIB_ClarkInv_SF_F32  SFunctionDeploymentMode=off  EnableBusSupport=off
  copyright : Subsystem
      mask Display:
      | text(10,90,'FILE:');text(10,75,'DESRIPTION:')
      | text(10,60,'COPYRIGHT:')
      | text(10,45,'VERSION:')
      | text(10,30,'DATE:')
  copyright2 : Subsystem
      mask Display:
      | text(10,90,'GMCLIB_ClarkInv_BAM_F32.mdl');text(10,75,'Inverse Clarke transformation');text(10,60,'NXP')
      | text(10,45,'0.1');text(10,30,'30-Aug-2011');
  logo : Subsystem
      mask Display: image(imread('logo.jpg'))
  f32A : Outport
  f32B : Outport  Port=2
  f32C : Outport  Port=3
  wires:
  GMCLIB_ClarkInv_SF_F32/3 -> f32C/1
  GMCLIB_ClarkInv_SF_F32/2 -> f32B/1
  GMCLIB_ClarkInv_SF_F32/1 -> f32A/1
  f32Beta/1 -> GMCLIB_ClarkInv_SF_F32/2
  f32Alpha/1 -> GMCLIB_ClarkInv_SF_F32/1

== system ammclib_bam_s32k11x/GMCLIB/bam_f32/GMCLIB_Clark_F32 ==
  note: ---------------------------------------------------------------------------------------------------------------------------------------------------------------------------------------------------
  f32A : Inport
  f32B : Inport  Port=2
  f32C : Inport  Port=3
  GMCLIB_Clark_SF_F32 : S-Function  FunctionName=GMCLIB_Clark_SF_F32  SFunctionDeploymentMode=off  EnableBusSupport=off
  copyright : Subsystem
      mask Display:
      | text(10,90,'FILE:');text(10,75,'DESRIPTION:')
      | text(10,60,'COPYRIGHT:')
      | text(10,45,'VERSION:')
      | text(10,30,'DATE:')
  copyright2 : Subsystem
      mask Display:
      | text(10,90,'GMCLIB_Clark_BAM_F32.mdl');text(10,75,'Clarke transformation.');text(10,60,'NXP')
      | text(10,45,'0.1');text(10,30,'29-Aug-2011');
  logo : Subsystem
      mask Display: image(imread('logo.jpg'))
  f32Alpha : Outport
  f32Beta : Outport  Port=2
  wires:
  GMCLIB_Clark_SF_F32/2 -> f32Beta/1
  GMCLIB_Clark_SF_F32/1 -> f32Alpha/1
  f32C/1 -> GMCLIB_Clark_SF_F32/3
  f32B/1 -> GMCLIB_Clark_SF_F32/2
  f32A/1 -> GMCLIB_Clark_SF_F32/1

== system ammclib_bam_s32k11x/GMCLIB/bam_f32/GMCLIB_DecouplingPMSM_F32 ==
  note: ---------------------------------------------------------------------------------------------------------------------------------------------------------------------------------------------------
  f32Ud : Inport
  f32Uq : Inport  Port=2
  f32Id : Inport  Port=3
  f32Iq : Inport  Port=4
  f32AngVel : Inport  Port=5
  GMCLIB_DecouplingPMSM_SF_F32 : S-Function  FunctionName=GMCLIB_DecouplingPMSM_SF_F32  Parameters=f32Kd,s16KdShift,f32Kq,s16KqShift  SFunctionDeploymentMode=off  EnableBusSupport=off
  copyright : Subsystem
      mask Display:
      | text(10,90,'FILE:');text(10,75,'DESRIPTION:')
      | text(10,60,'COPYRIGHT:')
      | text(10,45,'VERSION:')
      | text(10,30,'DATE:')
  copyright2 : Subsystem
      mask Display:
      | text(10,90,'GMCLIB_DecouplingPMSM_BAM_F32.mdl');text(10,75,'Decoupling of d and q axis of PMSM model.');text(10,60,'NXP')
      | text(10,45,'0.1');text(10,30,'14-Sep-2011');
  logo : Subsystem
      mask Display: image(imread('logo.jpg'))
  f32UdDec : Outport
  f32UqDec : Outport  Port=2
  wires:
  GMCLIB_DecouplingPMSM_SF_F32/2 -> f32UqDec/1
  GMCLIB_DecouplingPMSM_SF_F32/1 -> f32UdDec/1
  f32AngVel/1 -> GMCLIB_DecouplingPMSM_SF_F32/5
  f32Iq/1 -> GMCLIB_DecouplingPMSM_SF_F32/4
  f32Id/1 -> GMCLIB_DecouplingPMSM_SF_F32/3
  f32Uq/1 -> GMCLIB_DecouplingPMSM_SF_F32/2
  f32Ud/1 -> GMCLIB_DecouplingPMSM_SF_F32/1

== system ammclib_bam_s32k11x/GMCLIB/bam_f32/GMCLIB_ElimDcBusRip_F32 ==
  note: ---------------------------------------------------------------------------------------------------------------------------------------------------------------------------------------------------
  f32Alpha : Inport
  f32Beta : Inport  Port=2
  f32ArgDcBusMsr : Inport  Port=3
  GMCLIB_ElimDcBusRip_SF : S-Function  FunctionName=GMCLIB_ElimDcBusRip_SF_F32  Parameters=f32ModIndex  SFunctionDeploymentMode=off  EnableBusSupport=off
  copyright : Subsystem
      mask Display: text(10,90,'FILE:');text(10,75,'DESRIPTION:');text(10,60,'COPYRIGHT:');text(10,45,'VERSION:');text(10,30,'DATE:')
  copyright2 : Subsystem
      mask Display: text(10,90,'GMCLIB_ElimDcBusRip_BAM_F32.mdl');text(10,75,'DC Bus voltage ripple elimination function.');text(10,60,'NXP');text(10,45,'0.1');text(10,30,'12-Jun-2015');
  logo : Subsystem
      mask Display: image(imread('logo.jpg'))
  f32AlphaOut : Outport
  f32BetaOut : Outport  Port=2
  wires:
  GMCLIB_ElimDcBusRip_SF/2 -> f32BetaOut/1
  GMCLIB_ElimDcBusRip_SF/1 -> f32AlphaOut/1
  f32ArgDcBusMsr/1 -> GMCLIB_ElimDcBusRip_SF/3
  f32Beta/1 -> GMCLIB_ElimDcBusRip_SF/2
  f32Alpha/1 -> GMCLIB_ElimDcBusRip_SF/1

== system ammclib_bam_s32k11x/GMCLIB/bam_f32/GMCLIB_ParkInv_F32 ==
  note: ---------------------------------------------------------------------------------------------------------------------------------------------------------------------------------------------------
  f32D : Inport
  f32Q : Inport  Port=2
  f32Sin : Inport  Port=3
  f32Cos : Inport  Port=4
  GMCLIB_ParkInv_SF : S-Function  FunctionName=GMCLIB_ParkInv_SF_F32  SFunctionDeploymentMode=off  EnableBusSupport=off
  copyright : Subsystem
      mask Display:
      | text(10,90,'FILE:');text(10,75,'DESRIPTION:')
      | text(10,60,'COPYRIGHT:')
      | text(10,45,'VERSION:')
      | text(10,30,'DATE:')
  copyright2 : Subsystem
      mask Display:
      | text(10,90,'GMCLIB_ParkInv_BAM_F32.mdl');text(10,75,'Inverse Park transformation.');text(10,60,'Freescale')
      | text(10,45,'0.1');text(10,30,'19-Sep-2011');
  logo : Subsystem
      mask Display: image(imread('logo.jpg'))
  f32Alpha : Outport
  f32Beta : Outport  Port=2
  wires:
  GMCLIB_ParkInv_SF/2 -> f32Beta/1
  GMCLIB_ParkInv_SF/1 -> f32Alpha/1
  f32Cos/1 -> GMCLIB_ParkInv_SF/4
  f32Sin/1 -> GMCLIB_ParkInv_SF/3
  f32Q/1 -> GMCLIB_ParkInv_SF/2
  f32D/1 -> GMCLIB_ParkInv_SF/1

== system ammclib_bam_s32k11x/GMCLIB/bam_f32/GMCLIB_Park_F32 ==
  note: ---------------------------------------------------------------------------------------------------------------------------------------------------------------------------------------------------
  f32Alpha : Inport
  f32Beta : Inport  Port=2
  f32Sin : Inport  Port=3
  f32Cos : Inport  Port=4
  GMCLIB_Park_SF : S-Function  FunctionName=GMCLIB_Park_SF_F32  SFunctionDeploymentMode=off  EnableBusSupport=off
  copyright : Subsystem
      mask Display:
      | text(10,90,'FILE:');text(10,75,'DESRIPTION:')
      | text(10,60,'COPYRIGHT:')
      | text(10,45,'VERSION:')
      | text(10,30,'DATE:')
  copyright2 : Subsystem
      mask Display:
      | text(10,90,'GMCLIB_Park_BAM_F32.mdl');text(10,75,'Park transformation.');text(10,60,'NXP')
      | text(10,45,'0.1');text(10,30,'19-Sep-2011');
  logo : Subsystem
      mask Display: image(imread('logo.jpg'))
  f32D : Outport
  f32Q : Outport  Port=2
  wires:
  GMCLIB_Park_SF/2 -> f32Q/1
  GMCLIB_Park_SF/1 -> f32D/1
  f32Cos/1 -> GMCLIB_Park_SF/4
  f32Sin/1 -> GMCLIB_Park_SF/3
  f32Beta/1 -> GMCLIB_Park_SF/2
  f32Alpha/1 -> GMCLIB_Park_SF/1

== system ammclib_bam_s32k11x/GMCLIB/bam_f32/GMCLIB_PwmIct_F32 ==
  note: ---------------------------------------------------------------------------------------------------------------------------------------------------------------------------------------------------
  f32In1 : Inport
  f32In2 : Inport  Port=2
  GMCLIB_PwmIct_SF : S-Function  FunctionName=GMCLIB_PwmIct_SF_F32  SFunctionDeploymentMode=off  EnableBusSupport=off
  copyright : Subsystem
      mask Display: text(10,90,'FILE:');text(10,75,'DESRIPTION:');text(10,60,'COPYRIGHT:');text(10,45,'VERSION:');text(10,30,'DATE:')
  copyright2 : Subsystem
      mask Display: text(10,90,'GMCLIB_PwmIct_BAM_F32.mdl');text(10,75,'General Sinusoidal PWM.');text(10,60,'NXP');text(10,45,'1.0');text(10,30,'05-Apr-2019');
  logo : Subsystem
      mask Display: image(imread('logo.jpg'))
  f32Out1 : Outport
  f32Out2 : Outport  Port=2
  f32Out3 : Outport  Port=3
  u32Sector : Outport  Port=4
  wires:
  f32In1/1 -> GMCLIB_PwmIct_SF/1
  f32In2/1 -> GMCLIB_PwmIct_SF/2
  GMCLIB_PwmIct_SF/1 -> f32Out1/1
  GMCLIB_PwmIct_SF/2 -> f32Out2/1
  GMCLIB_PwmIct_SF/3 -> f32Out3/1
  GMCLIB_PwmIct_SF/4 -> u32Sector/1

== system ammclib_bam_s32k11x/GMCLIB/bam_f32/GMCLIB_SvmStd_F32 ==
  note: ---------------------------------------------------------------------------------------------------------------------------------------------------------------------------------------------------
  f32In1 : Inport
  f32In2 : Inport  Port=2
  GMCLIB_SvmStd_SF : S-Function  FunctionName=GMCLIB_SvmStd_SF_F32  SFunctionDeploymentMode=off  EnableBusSupport=off
  copyright : Subsystem
      mask Display:
      | text(10,90,'FILE:');text(10,75,'DESRIPTION:')
      | text(10,60,'COPYRIGHT:')
      | text(10,45,'VERSION:')
      | text(10,30,'DATE:')
  copyright2 : Subsystem
      mask Display:
      | text(10,90,'GMCLIB_SvmStd_BAM_F32.mdl');text(10,75,'Standard Space Vector Modulation.');text(10,60,'NXP')
      | text(10,45,'0.1');text(10,30,'26-Sep-2011');
  logo : Subsystem
      mask Display: image(imread('logo.jpg'))
  f32Out1 : Outport
  f32Out2 : Outport  Port=2
  f32Out3 : Outport  Port=3
  u32Sector : Outport  Port=4
  wires:
  GMCLIB_SvmStd_SF/4 -> u32Sector/1
  GMCLIB_SvmStd_SF/3 -> f32Out3/1
  GMCLIB_SvmStd_SF/2 -> f32Out2/1
  GMCLIB_SvmStd_SF/1 -> f32Out1/1
  f32In2/1 -> GMCLIB_SvmStd_SF/2
  f32In1/1 -> GMCLIB_SvmStd_SF/1

== system ammclib_bam_s32k11x/GMCLIB/bam_f32/GMCLIB_SvmU0n_F32 ==
  note: ---------------------------------------------------------------------------------------------------------------------------------------------------------------------------------------------------
  f32In1 : Inport
  f32In2 : Inport  Port=2
  GMCLIB_SvmU0n_SF : S-Function  FunctionName=GMCLIB_SvmU0n_SF_F32  SFunctionDeploymentMode=off  EnableBusSupport=off
  copyright : Subsystem
      mask Display: text(10,90,'FILE:');text(10,75,'DESRIPTION:');text(10,60,'COPYRIGHT:');text(10,45,'VERSION:');text(10,30,'DATE:')
  copyright2 : Subsystem
      mask Display: text(10,90,'GMCLIB_SvmU0n_BAM_F32.mdl');text(10,75,'Standard Space Vector Modulation.');text(10,60,'NXP');text(10,45,'0.1');text(10,30,'02-Apr-2019');
  logo : Subsystem
      mask Display: image(imread('logo.jpg'))
  f32Out1 : Outport
  f32Out2 : Outport  Port=2
  f32Out3 : Outport  Port=3
  u32Sector : Outport  Port=4
  wires:
  f32In1/1 -> GMCLIB_SvmU0n_SF/1
  f32In2/1 -> GMCLIB_SvmU0n_SF/2
  GMCLIB_SvmU0n_SF/1 -> f32Out1/1
  GMCLIB_SvmU0n_SF/2 -> f32Out2/1
  GMCLIB_SvmU0n_SF/3 -> f32Out3/1
  GMCLIB_SvmU0n_SF/4 -> u32Sector/1

== system ammclib_bam_s32k11x/MLIB/bam_f16/MLIB_AbsSat_F16 ==
  note: ---------------------------------------------------------------------------------------------------------------------------------------------------------------------------------------------------
  f16In : Inport
  MLIB_AbsSat_SF : S-Function  FunctionName=MLIB_AbsSat_SF_F16  SFunctionDeploymentMode=off  EnableBusSupport=off
  copyright : Subsystem
      mask Display: text(10,90,'FILE:');text(10,75,'DESRIPTION:')text(10,60,'COPYRIGHT:')text(10,45,'VERSION:')text(10,30,'DATE:')
  copyright2 : Subsystem
      mask Display: text(10,90,'MLIB_AbsSat_BAM_F16.mdl');text(10,75,'Absolute value of input parameter saturated if necessary.');text(10,60,'NXP')text(10,45,'0.1');text(10,30,'19-Aug-2011');
  logo : Subsystem
      mask Display: image(imread('logo.jpg'))
  f16Out : Outport
  wires:
  MLIB_AbsSat_SF/1 -> f16Out/1
  f16In/1 -> MLIB_AbsSat_SF/1

== system ammclib_bam_s32k11x/MLIB/bam_f16/MLIB_Abs_F16 ==
  note: ---------------------------------------------------------------------------------------------------------------------------------------------------------------------------------------------------
  f16In : Inport
  MLIB_Abs_SF : S-Function  FunctionName=MLIB_Abs_SF_F16  SFunctionDeploymentMode=off  EnableBusSupport=off
  copyright : Subsystem
      mask Display: text(10,90,'FILE:');text(10,75,'DESRIPTION:')text(10,60,'COPYRIGHT:')text(10,45,'VERSION:')text(10,30,'DATE:')
  copyright2 : Subsystem
      mask Display: text(10,90,'MLIB_Abs_BAM_F16.mdl');text(10,75,'Absolute value of input parameter.');text(10,60,'Freescale')text(10,45,'0.1');text(10,30,'20-Jan-2012');
  logo : Subsystem
      mask Display: image(imread('logo.jpg'))
  f16Out : Outport
  wires:
  MLIB_Abs_SF/1 -> f16Out/1
  f16In/1 -> MLIB_Abs_SF/1
